simulink model "intercambiador_calor"  (R2020a)
settings: Solver=VariableStepAuto  StartTime=0.0  StopTime=10  RelTol=1e-3
values from neighbouring files (symbols this model uses):
  Cc = 4180    [Codigo_Intercambiador_calor.m]
  Ch = 4180    [Codigo_Intercambiador_calor.m]
  Fc = 0.05    [Codigo_Intercambiador_calor.m]
  Fh = 0.11    [Codigo_Intercambiador_calor.m]
  k = 2*10^5    (= 200000)    [Codigo_Intercambiador_calor.m]
  pc = 1000    [Codigo_Intercambiador_calor.m]
  ph = 1000    [Codigo_Intercambiador_calor.m]
  Tc0 = 20    [Codigo_Intercambiador_calor.m]
  Th0 = 90    [Codigo_Intercambiador_calor.m]
  Vc = 0.2    [Codigo_Intercambiador_calor.m]
  Vh = 0.2    [Codigo_Intercambiador_calor.m]
undefined symbols (not defined in the file or in its folder): temp_cold, temp_hot
settings Model: Creator=cral-2204  LastModifiedBy=cral-2204

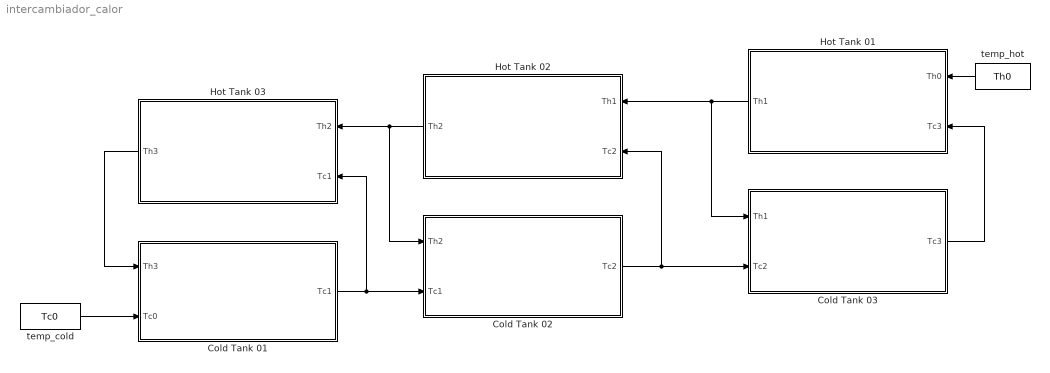
== system intercambiador_calor ==
  Cold Tank 01 : Subsystem
  Cold Tank 02 : Subsystem
  Cold Tank 03 : Subsystem
  Hot Tank 01 : Subsystem
  Hot Tank 02 : Subsystem
  Hot Tank 03 : Subsystem
  temp_cold : Constant  Value=Tc0
  temp_hot : Constant  Value=Th0
  wires:
  Cold Tank 02/1(Tc2) -> Cold Tank 03/2(Tc2), Hot Tank 02/2(Tc2)
  Cold Tank 01/1(Tc1) -> Cold Tank 02/2(Tc1), Hot Tank 03/2(Tc1)
  temp_cold/1 -> Cold Tank 01/2(Tc0)
  Hot Tank 01/1(Th1) -> Cold Tank 03/1(Th1), Hot Tank 02/1(Th1)
  temp_hot/1 -> Hot Tank 01/1(Th0)
  Cold Tank 03/1(Tc3) -> Hot Tank 01/2(Tc3)
  Hot Tank 02/1(Th2) -> Cold Tank 02/1(Th2), Hot Tank 03/1(Th2)
  Hot Tank 03/1(Th3) -> Cold Tank 01/1(Th3)

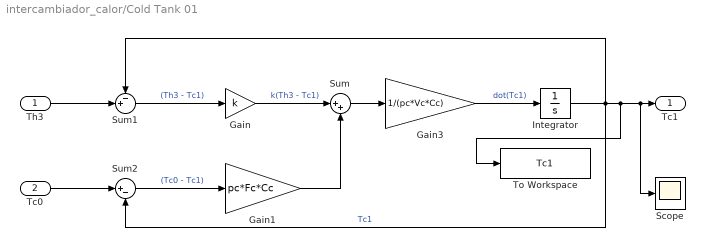
== system intercambiador_calor/Cold Tank 01 ==
  Th3 : Inport
  Tc0 : Inport  Port=2
  Gain : Gain  Gain=k
  Gain1 : Gain  Gain=pc*Fc*Cc
  Gain3 : Gain  Gain=1/(pc*Vc*Cc)
  Integrator : Integrator  InitialCondition=temp_cold
  Scope : Scope
  Sum : Sum  Inputs=|++
  Sum1 : Sum  Inputs=-+|
  Sum2 : Sum  Inputs=|+-
  To Workspace : ToWorkspace  VariableName=Tc1  SaveFormat=Structure With Time  SampleTime=-1
  Tc1 : Outport
  wires:
  Th3/1 -> Sum1/2
  Gain3/1 -> Integrator/1  "dot(Tc1)"
  Gain/1 -> Sum/1  "k(Th3 - Tc1)"
  Sum/1 -> Gain3/1
  Sum2/1 -> Gain1/1  "(Tc0 - Tc1)"
  Integrator/1 -> Scope/1, Tc1/1, To Workspace/1, Sum2/2, Sum1/1  "Tc1"
  Gain1/1 -> Sum/2
  Sum1/1 -> Gain/1  "(Th3 - Tc1)"
  Tc0/1 -> Sum2/1

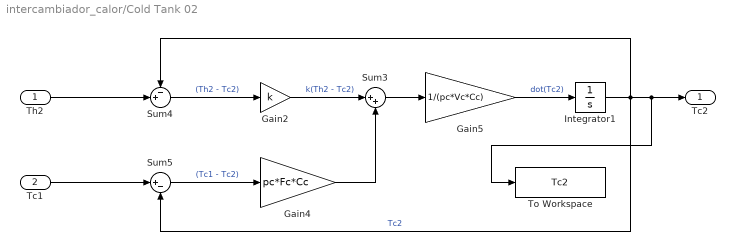
== system intercambiador_calor/Cold Tank 02 ==
  Th2 : Inport
  Tc1 : Inport  Port=2
  Gain2 : Gain  Gain=k
  Gain4 : Gain  Gain=pc*Fc*Cc
  Gain5 : Gain  Gain=1/(pc*Vc*Cc)
  Integrator1 : Integrator  InitialCondition=temp_cold
  Sum3 : Sum  Inputs=|++
  Sum4 : Sum  Inputs=-+|
  Sum5 : Sum  Inputs=|+-
  To Workspace : ToWorkspace  VariableName=Tc2  SaveFormat=Structure With Time  SampleTime=-1
  Tc2 : Outport
  wires:
  Gain5/1 -> Integrator1/1  "dot(Tc2)"
  Gain4/1 -> Sum3/2
  Sum4/1 -> Gain2/1  "(Th2 - Tc2)"
  Integrator1/1 -> To Workspace/1, Tc2/1, Sum5/2, Sum4/1  "Tc2"
  Sum3/1 -> Gain5/1
  Th2/1 -> Sum4/2
  Gain2/1 -> Sum3/1  "k(Th2 - Tc2)"
  Tc1/1 -> Sum5/1
  Sum5/1 -> Gain4/1  "(Tc1 - Tc2)"

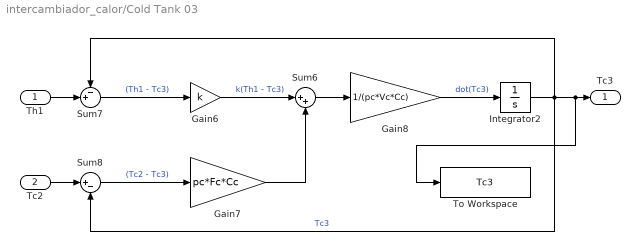
== system intercambiador_calor/Cold Tank 03 ==
  Th1 : Inport
  Tc2 : Inport  Port=2
  Gain6 : Gain  Gain=k
  Gain7 : Gain  Gain=pc*Fc*Cc
  Gain8 : Gain  Gain=1/(pc*Vc*Cc)
  Integrator2 : Integrator  InitialCondition=temp_cold
  Sum6 : Sum  Inputs=|++
  Sum7 : Sum  Inputs=-+|
  Sum8 : Sum  Inputs=|+-
  To Workspace : ToWorkspace  VariableName=Tc3  SaveFormat=Structure With Time  SampleTime=-1
  Tc3 : Outport
  wires:
  Sum8/1 -> Gain7/1  "(Tc2 - Tc3)"
  Gain8/1 -> Integrator2/1  "dot(Tc3)"
  Sum7/1 -> Gain6/1  "(Th1 - Tc3)"
  Tc2/1 -> Sum8/1
  Sum6/1 -> Gain8/1
  Th1/1 -> Sum7/2
  Gain7/1 -> Sum6/2
  Gain6/1 -> Sum6/1  "k(Th1 - Tc3)"
  Integrator2/1 -> To Workspace/1, Tc3/1, Sum8/2, Sum7/1  "Tc3"

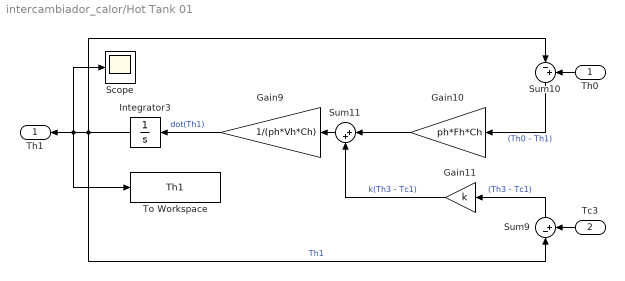
== system intercambiador_calor/Hot Tank 01 ==
  Th0 : Inport
  Tc3 : Inport  Port=2
  Gain10 : Gain  Gain=ph*Fh*Ch
  Gain11 : Gain  Gain=k
  Gain9 : Gain  Gain=1/(ph*Vh*Ch)
  Integrator3 : Integrator  InitialCondition=temp_hot
  Scope : Scope
  Sum10 : Sum  Inputs=|-+
  Sum11 : Sum  Inputs=|++
  Sum9 : Sum  Inputs=|-+
  To Workspace : ToWorkspace  VariableName=Th1  SaveFormat=Structure With Time  SampleTime=-1
  Th1 : Outport
  wires:
  Sum10/1 -> Gain10/1  "(Th0 - Th1)"
  Th0/1 -> Sum10/2
  Gain10/1 -> Sum11/1
  Gain11/1 -> Sum11/2  "k(Th3 - Tc1)"
  Gain9/1 -> Integrator3/1  "dot(Th1)"
  Integrator3/1 -> To Workspace/1, Th1/1, Scope/1, Sum10/1, Sum9/1  "Th1"
  Sum11/1 -> Gain9/1
  Sum9/1 -> Gain11/1  "(Th3 - Tc1)"
  Tc3/1 -> Sum9/2

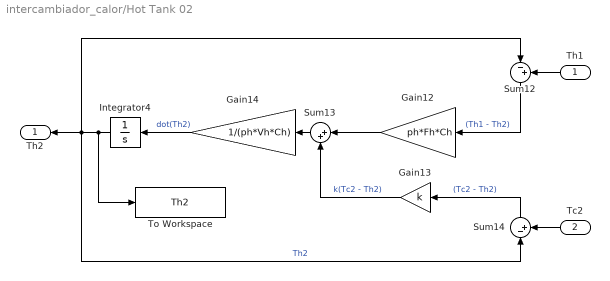
== system intercambiador_calor/Hot Tank 02 ==
  Th1 : Inport
  Tc2 : Inport  Port=2
  Gain12 : Gain  Gain=ph*Fh*Ch
  Gain13 : Gain  Gain=k
  Gain14 : Gain  Gain=1/(ph*Vh*Ch)
  Integrator4 : Integrator  InitialCondition=temp_hot
  Sum12 : Sum  Inputs=|-+
  Sum13 : Sum  Inputs=|++
  Sum14 : Sum  Inputs=|-+
  To Workspace : ToWorkspace  VariableName=Th2  SaveFormat=Structure With Time  SampleTime=-1
  Th2 : Outport
  wires:
  Sum12/1 -> Gain12/1  "(Th1 - Th2)"
  Gain14/1 -> Integrator4/1  "dot(Th2)"
  Integrator4/1 -> To Workspace/1, Th2/1, Sum14/1, Sum12/1  "Th2"
  Gain12/1 -> Sum13/1
  Gain13/1 -> Sum13/2  "k(Tc2 - Th2)"
  Sum13/1 -> Gain14/1
  Sum14/1 -> Gain13/1  "(Tc2 - Th2)"
  Tc2/1 -> Sum14/2
  Th1/1 -> Sum12/2

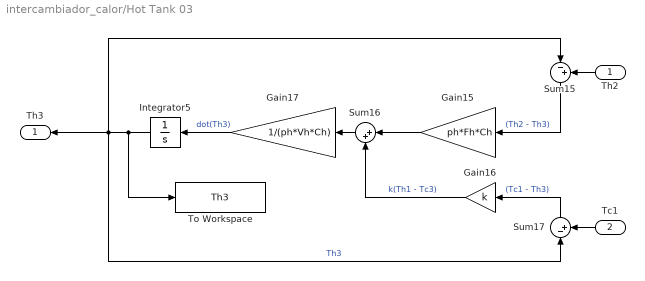
== system intercambiador_calor/Hot Tank 03 ==
  Th2 : Inport
  Tc1 : Inport  Port=2
  Gain15 : Gain  Gain=ph*Fh*Ch
  Gain16 : Gain  Gain=k
  Gain17 : Gain  Gain=1/(ph*Vh*Ch)
  Integrator5 : Integrator  InitialCondition=temp_hot
  Sum15 : Sum  Inputs=|-+
  Sum16 : Sum  Inputs=|++
  Sum17 : Sum  Inputs=|-+
  To Workspace : ToWorkspace  VariableName=Th3  SaveFormat=Structure With Time  SampleTime=-1
  Th3 : Outport
  wires:
  Gain17/1 -> Integrator5/1  "dot(Th3)"
  Sum15/1 -> Gain15/1  "(Th2 - Th3)"
  Integrator5/1 -> To Workspace/1, Sum15/1, Th3/1, Sum17/1  "Th3"
  Th2/1 -> Sum15/2
  Gain15/1 -> Sum16/1
  Sum17/1 -> Gain16/1  "(Tc1 - Th3)"
  Sum16/1 -> Gain17/1
  Gain16/1 -> Sum16/2  "k(Th1 - Tc3)"
  Tc1/1 -> Sum17/2
